simulink model "Modular_Model_New_Board_Enes"  (R2018a)
settings: Solver=VariableStepAuto  StartTime=0.0  StopTime=Tfinal  FixedStep=SampleTime*1e-2  MinStep=SampleTime*1e-2  RelTol=1e-3
values from neighbouring files (symbols this model uses):
  C1A = 5e-6    (= 5e-06)    [InverterMFile.m]    (also in sim_param_new_board.m)
  C1B = 5e-6    (= 5e-06)    [InverterMFile.m]    (also in sim_param_new_board.m)
  C1C = 5e-6    (= 5e-06)    [InverterMFile.m]    (also in sim_param_new_board.m)
  ESLA = 19e-15    (= 1.9e-14)    [sim_param_new_board.m]
  ESLB = 19e-15    (= 1.9e-14)    [sim_param_new_board.m]
  ESLC = 19e-15    (= 1.9e-14)    [sim_param_new_board.m]
  ESRA = 21.1e-15    (= 2.11e-14)    [sim_param_new_board.m]
  ESRB = 21.1e-15    (= 2.11e-14)    [sim_param_new_board.m]
  ESRC = 21.1e-15    (= 2.11e-14)    [sim_param_new_board.m]
  ffund = 50    [InverterMFile.m]    (also in mathematicalModelParam.m; sim_param_new_board.m)
  LABBot = 10.20e-9    (= 1.02e-08)    [sim_param_new_board.m]
  LABot = 20.25e-9    (= 2.025e-08)    [sim_param_new_board.m]
  LABTop = 18.30e-9    (= 1.83e-08)    [sim_param_new_board.m]
  LAMid = 01.30e-9    (= 1.3e-09)    [sim_param_new_board.m]
  LATop = 03.40e-9    (= 3.4e-09)    [sim_param_new_board.m]
  LBBot = 20.38e-9    (= 2.038e-08)    [sim_param_new_board.m]
  LBCBot = 11.14e-9    (= 1.114e-08)    [sim_param_new_board.m]
  LBCTop = 21.84e-9    (= 2.184e-08)    [sim_param_new_board.m]
  LBMid = 01.30e-9    (= 1.3e-09)    [sim_param_new_board.m]
  LBTop = 03.38e-9    (= 3.38e-09)    [sim_param_new_board.m]
  LCBot = 20.94e-9    (= 2.094e-08)    [sim_param_new_board.m]
  LCMid = 01.30e-9    (= 1.3e-09)    [sim_param_new_board.m]
  LCTop = 03.41e-9    (= 3.41e-09)    [sim_param_new_board.m]
  Ld = 0.9e-9    (= 9e-10)    [InverterMFile.m]    (also in sim_param_new_board.m)
  Lin = Lload1    [InverterMFile.m]    (also in sim_param_new_board.m)
  Lload1 = Xload1/(2*pi*ffund)    [InverterMFile.m]    (also in sim_param_new_board.m)
  Ls = 0.9e-9    (= 9e-10)    [InverterMFile.m]    (also in sim_param_new_board.m)
  ModulationIndex1 = 0.9    [InverterMFile.m]    (also in sim_param_new_board.m)
  Module1Phase = 0    [InverterMFile.m]    (also in sim_param_new_board.m)
  NEG1 = 100e-15    (= 1e-13)    [InverterMFile.m]    (also in sim_param_new_board.m)
  POS1 = 100e-15    (= 1e-13)    [InverterMFile.m]    (also in sim_param_new_board.m)
  RABBot = 10.20e-9    (= 1.02e-08)    [sim_param_new_board.m]
  RABot = 20.25e-9    (= 2.025e-08)    [sim_param_new_board.m]
  RABTop = 18.30e-9    (= 1.83e-08)    [sim_param_new_board.m]
  RAMid = 01.30e-9    (= 1.3e-09)    [sim_param_new_board.m]
  RATop = 03.40e-9    (= 3.4e-09)    [sim_param_new_board.m]
  RBBot = 20.38e-9    (= 2.038e-08)    [sim_param_new_board.m]
  RBCBot = 11.14e-9    (= 1.114e-08)    [sim_param_new_board.m]
  RBCTop = 21.84e-9    (= 2.184e-08)    [sim_param_new_board.m]
  RBMid = 01.30e-9    (= 1.3e-09)    [sim_param_new_board.m]
  RBTop = 03.38e-9    (= 3.38e-09)    [sim_param_new_board.m]
  RCBot = 20.94e-9    (= 2.094e-08)    [sim_param_new_board.m]
  RCMid = 01.30e-9    (= 1.3e-09)    [sim_param_new_board.m]
  RCTop = 03.41e-9    (= 3.41e-09)    [sim_param_new_board.m]
  Rin = 10    [InverterMFile.m]    (also in sim_param_new_board.m)
  Rload1 = Z1*PF    [InverterMFile.m]    (also in sim_param_new_board.m)
  Vin = Vdc + Idc*Rin    (= 418.148148148)    [InverterMFile.m]    (also in sim_param_new_board.m = 147.040202596)
  Vmodule = 270    [InverterMFile.m]    (also in sim_param_new_board.m)
  VpulseMax = 6    [InverterMFile.m]    (also in sim_param_new_board.m)
  VpulseMin = -3    [InverterMFile.m]    (also in sim_param_new_board.m)
libraries: powerlib x80, simulink x12, powerlib_meascontrol x4
settings Model: SimulationMode=accelerator  Creator=Furkan  LastModifiedBy=enes_
settings DataIOCC: SaveOutput=off  SignalLogging=off  DSMLogging=off  SaveTime=off
settings OptimizationCC: LifeSpan=inf
settings DebuggingCC: SFExecutionAtInitializationDiag=none
settings CodeAppCC: StateflowObjectComments=on
settings SimscapeCC: SimscapeNormalizeSystem=off

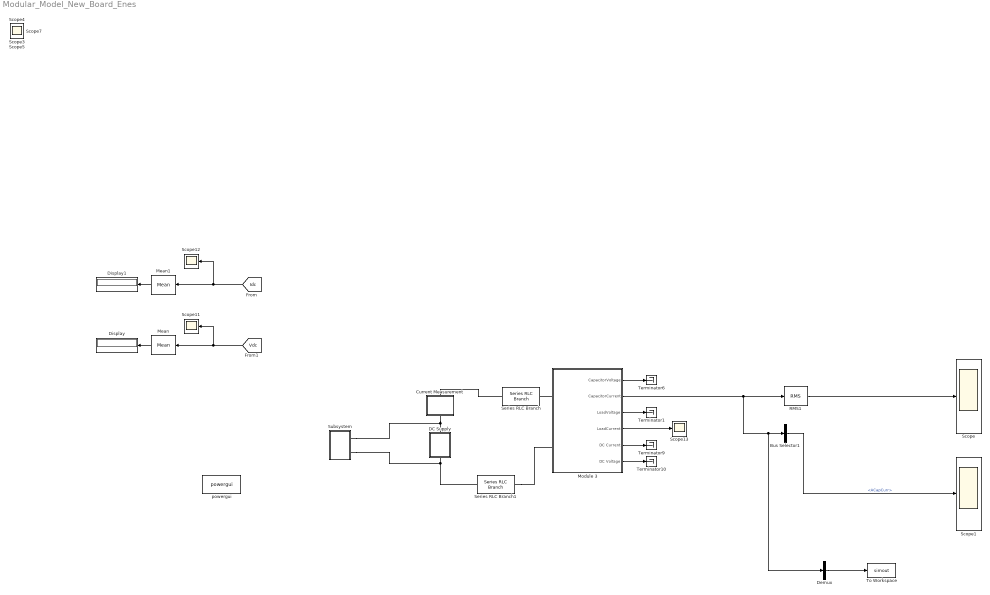
== system Modular_Model_New_Board_Enes ==
  Bus Selector1 : BusSelector  OutputSignals=ACapCurr
  Current Measurement : Subsystem
  DC Supply : Subsystem
  Demux : Demux  Outputs=3
  Display : Display
  Display1 : Display
  Mean : powerlib_meascontrol/Measurements/Mean  Freq=ffund  Vinit=0  Ts=0
  Mean1 : powerlib_meascontrol/Measurements/Mean  Freq=ffund  Vinit=0  Ts=0
  Module 3 : Subsystem
  RMS1 : powerlib_meascontrol/Measurements/RMS  TrueRMS=on  Freq=40000  RMSInit=0  Ts=0
  Scope : Scope  NumInputPorts=3
  Scope1 : Scope  NumInputPorts=3
  Scope{3..5,7,11..13} (7 alike) : Scope
  Series RLC Branch : powerlib/Elements/Series RLC Branch  LConnTagsString=__new0  RConnTagsString=__new0  BranchType=L  Resistance=1  Inductance=POS1  SetiL0=off  InitialCurrent=0  Capacitance=1e-6  Setx0=off  InitialVoltage=0  Measurements=None
  Series RLC Branch1 : powerlib/Elements/Series RLC Branch  LConnTagsString=__new0  RConnTagsString=__new0  BranchType=L  Resistance=1  Inductance=NEG1  SetiL0=off  InitialCurrent=0  Capacitance=1e-6  Setx0=off  InitialVoltage=0  Measurements=None
  Subsystem : Subsystem
  Terminator{1,6,9..10} (4 alike) : Terminator
  To Workspace : ToWorkspace  VariableName=simout  SaveFormat=Timeseries  SampleTime=-1
  powergui : powerlib/powergui  Priority=1  SimulationMode=Discrete  SampleTime=5e-6  frequency=60  Iterations=50  frequencyindice=0  Pbase=100e6  ErrMax=1e-4  UnitsV=kV  UnitsW=MW  buscounter=0  FunctionMessages=off  echomessages=off  EnableUseOfTLC=off  CurrentSourceSwitches=off  DisableSnubberDevices=off  DisableRonSwitches=off  DisableVfSwitches=off  DisplayEquations=off  SolverType=Tustin/Backward Euler (TBE)  Interpol=off  ExternalGateDelay=off  methode=off  Ts=100  x0status=blocks  SPID=off  SwTol=0  HookPort=off  RestoreLinks=warning  ResistiveCurrentMeasurement=off  Frange=[0:2:500]  Ylog=off  Xlog=on  ShowGrid=off  save=off  variable=ZData  structure=0  ZoomFFT=off  StartTime=0.0  cycles=1  DisplayStyle=1  fundamental=60  FreqAxis=off  MaxFrequency=1000  frequencyindicesteady=1  RmsSteady=1  display=off
  wires:
  [Vdc] -> Mean/1, Scope11/1
  [Idc] -> Mean1/1, Scope12/1
  Module 3/1(CapacitorVoltage) -> Terminator6/1
  Module 3/2(CapacitorCurrent) -> Demux/1, Bus Selector1/1, RMS1/1
  Module 3/5(DC Current) -> Terminator9/1
  Module 3/6(DC Voltage) -> Terminator10/1
  RMS1/1 -> Scope/2
  Bus Selector1/1 -> Scope1/2  "<ACapCurr>"
  Mean/1 -> Display/1
  Mean1/1 -> Display1/1
  Module 3/3(LoadVoltage) -> Terminator1/1
  Module 3/4(LoadCurrent) -> Scope13/1
  Demux/2 -> To Workspace/1
  connections:
  DC Supply/LConn1 -- Series RLC Branch1/LConn1 -- Subsystem/LConn2
  Current Measurement/RConn1 -- DC Supply/RConn1 -- Subsystem/LConn1
  Module 3/LConn1 -- Series RLC Branch/RConn1
  Current Measurement/LConn1 -- Series RLC Branch/LConn1
  Series RLC Branch1/RConn1 -- Module 3/LConn2

== system Modular_Model_New_Board_Enes/Current Measurement ==
  Current Measurement : powerlib/Measurements/Current Measurement  PhasorSimulation=off  OutputType=Complex  PSBequivalent=0
  DC+ : PMIOPort  Side=Left
  i+ : PMIOPort  Port=2  Side=Right
  tag scope: Idc=global
  wires:
  Current Measurement/1 -> [Idc]
  connections:
  DC+/RConn1 -- Current Measurement/RConn1
  Current Measurement/LConn1 -- i+/RConn1

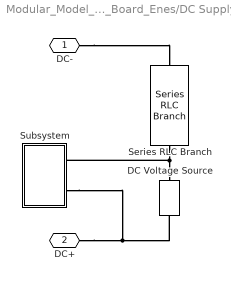
== system Modular_Model_New_Board_Enes/DC Supply ==
  DC Voltage Source : powerlib/Electrical Sources/DC Voltage Source  Amplitude=Vin  Measurements=None
  Series RLC Branch : powerlib/Elements/Series RLC Branch  LConnTagsString=__new0  RConnTagsString=__new0  BranchType=RL  Resistance=Rin  Inductance=Lin  SetiL0=off  InitialCurrent=0  Capacitance=1e-6  Setx0=off  InitialVoltage=0  Measurements=None
  Subsystem : Subsystem
  DC- : PMIOPort  Side=Left
  DC+ : PMIOPort  Port=2  Side=Right
  connections:
  DC-/RConn1 -- Series RLC Branch/RConn1
  DC+/RConn1 -- Subsystem/LConn2 -- DC Voltage Source/RConn1
  Series RLC Branch/LConn1 -- DC Voltage Source/LConn1 -- Subsystem/LConn1

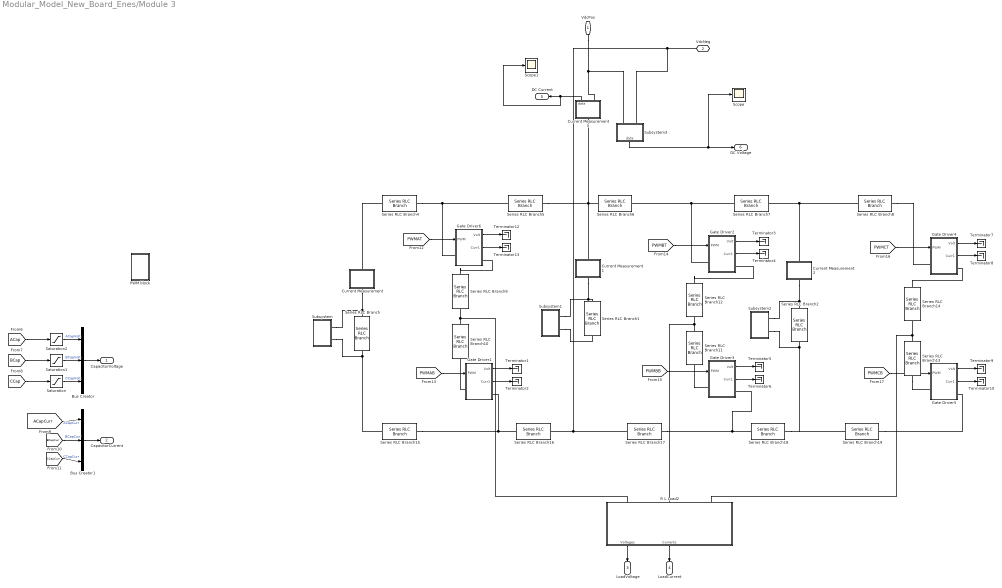
== system Modular_Model_New_Board_Enes/Module 3 ==
  Bus Creator : BusCreator  Inputs=3
  Bus Creator1 : BusCreator  Inputs=3
  Current Measurement : Subsystem
  Current Measurement1 : Subsystem
  Current Measurement2 : Subsystem
  Current Measurement3 : Subsystem
  Gate Driver1 : Subsystem
  Gate Driver2 : Subsystem
  Gate Driver3 : Subsystem
  Gate Driver4 : Subsystem
  Gate Driver5 : Subsystem
  Gate Driver6 : Subsystem
  PWM block : Subsystem
  R L Load2 : Subsystem
  Saturation : Saturate  UpperLimit=Vmodule*1.5  LowerLimit=-20
  Saturation1 : Saturate  UpperLimit=Vmodule*1.5  LowerLimit=-20
  Saturation2 : Saturate  UpperLimit=Vmodule*1.5  LowerLimit=-20
  Scope : Scope
  Scope1 : Scope
  Series RLC Branch : powerlib/Elements/Series RLC Branch  LConnTagsString=__new0  RConnTagsString=__new0  BranchType=RLC  Resistance=ESRA  Inductance=ESLA  SetiL0=off  InitialCurrent=0  Capacitance=C1A  Setx0=on  InitialVoltage=Vdc  Measurements=None
  Series RLC Branch1 : powerlib/Elements/Series RLC Branch  LConnTagsString=__new0  RConnTagsString=__new0  BranchType=RLC  Resistance=ESRB  Inductance=ESLB  SetiL0=off  InitialCurrent=0  Capacitance=C1B  Setx0=on  InitialVoltage=Vdc  Measurements=None
  Series RLC Branch10 : powerlib/Elements/Series RLC Branch  LConnTagsString=__new0  RConnTagsString=__new0  BranchType=RL  Resistance=RAMid/2  Inductance=LAMid/2  SetiL0=off  InitialCurrent=0  Capacitance=1e-6  Setx0=off  InitialVoltage=0  Measurements=None
  Series RLC Branch11 : powerlib/Elements/Series RLC Branch  LConnTagsString=__new0  RConnTagsString=__new0  BranchType=RL  Resistance=RBMid/2  Inductance=LBMid/2  SetiL0=off  InitialCurrent=0  Capacitance=1e-6  Setx0=off  InitialVoltage=0  Measurements=None
  Series RLC Branch12 : powerlib/Elements/Series RLC Branch  LConnTagsString=__new0  RConnTagsString=__new0  BranchType=RL  Resistance=RBMid/2  Inductance=LBMid/2  SetiL0=off  InitialCurrent=0  Capacitance=1e-6  Setx0=off  InitialVoltage=0  Measurements=None
  Series RLC Branch13 : powerlib/Elements/Series RLC Branch  LConnTagsString=__new0  RConnTagsString=__new0  BranchType=RL  Resistance=RCMid/2  Inductance=LCMid/2  SetiL0=off  InitialCurrent=0  Capacitance=1e-6  Setx0=off  InitialVoltage=0  Measurements=None
  Series RLC Branch14 : powerlib/Elements/Series RLC Branch  LConnTagsString=__new0  RConnTagsString=__new0  BranchType=RL  Resistance=RCMid/2  Inductance=LCMid/2  SetiL0=off  InitialCurrent=0  Capacitance=1e-6  Setx0=off  InitialVoltage=0  Measurements=None
  Series RLC Branch15 : powerlib/Elements/Series RLC Branch  LConnTagsString=__new0  RConnTagsString=__new0  BranchType=RL  Resistance=RABot  Inductance=LABot  SetiL0=off  InitialCurrent=0  Capacitance=1e-6  Setx0=off  InitialVoltage=0  Measurements=None
  Series RLC Branch16 : powerlib/Elements/Series RLC Branch  LConnTagsString=__new0  RConnTagsString=__new0  BranchType=RL  Resistance=RABBot  Inductance=LABBot  SetiL0=off  InitialCurrent=0  Capacitance=1e-6  Setx0=off  InitialVoltage=0  Measurements=None
  Series RLC Branch17 : powerlib/Elements/Series RLC Branch  LConnTagsString=__new0  RConnTagsString=__new0  BranchType=RL  Resistance=RBBot  Inductance=LBBot  SetiL0=off  InitialCurrent=0  Capacitance=1e-6  Setx0=off  InitialVoltage=0  Measurements=None
  Series RLC Branch18 : powerlib/Elements/Series RLC Branch  LConnTagsString=__new0  RConnTagsString=__new0  BranchType=RL  Resistance=RBCBot  Inductance=LBCBot  SetiL0=off  InitialCurrent=0  Capacitance=1e-6  Setx0=off  InitialVoltage=0  Measurements=None
  Series RLC Branch19 : powerlib/Elements/Series RLC Branch  LConnTagsString=__new0  RConnTagsString=__new0  BranchType=RL  Resistance=RCBot  Inductance=LCBot  SetiL0=off  InitialCurrent=0  Capacitance=1e-6  Setx0=off  InitialVoltage=0  Measurements=None
  Series RLC Branch2 : powerlib/Elements/Series RLC Branch  LConnTagsString=__new0  RConnTagsString=__new0  BranchType=RLC  Resistance=ESRC  Inductance=ESLC  SetiL0=off  InitialCurrent=0  Capacitance=C1C  Setx0=on  InitialVoltage=Vdc  Measurements=None
  Series RLC Branch4 : powerlib/Elements/Series RLC Branch  LConnTagsString=__new0  RConnTagsString=__new0  BranchType=RL  Resistance=RATop  Inductance=LATop  SetiL0=off  InitialCurrent=0  Capacitance=1e-6  Setx0=off  InitialVoltage=0  Measurements=None
  Series RLC Branch5 : powerlib/Elements/Series RLC Branch  LConnTagsString=__new0  RConnTagsString=__new0  BranchType=RL  Resistance=RABTop  Inductance=LABTop  SetiL0=off  InitialCurrent=0  Capacitance=1e-6  Setx0=off  InitialVoltage=0  Measurements=None
  Series RLC Branch6 : powerlib/Elements/Series RLC Branch  LConnTagsString=__new0  RConnTagsString=__new0  BranchType=RL  Resistance=RBTop  Inductance=LBTop  SetiL0=off  InitialCurrent=0  Capacitance=1e-6  Setx0=off  InitialVoltage=0  Measurements=None
  Series RLC Branch7 : powerlib/Elements/Series RLC Branch  LConnTagsString=__new0  RConnTagsString=__new0  BranchType=RL  Resistance=RBCTop  Inductance=LBCTop  SetiL0=off  InitialCurrent=0  Capacitance=1e-6  Setx0=off  InitialVoltage=0  Measurements=None
  Series RLC Branch8 : powerlib/Elements/Series RLC Branch  LConnTagsString=__new0  RConnTagsString=__new0  BranchType=RL  Resistance=RCTop  Inductance=LCTop  SetiL0=off  InitialCurrent=0  Capacitance=1e-6  Setx0=off  InitialVoltage=0  Measurements=None
  Series RLC Branch9 : powerlib/Elements/Series RLC Branch  LConnTagsString=__new0  RConnTagsString=__new0  BranchType=RL  Resistance=RAMid/2  Inductance=LAMid/2  SetiL0=off  InitialCurrent=0  Capacitance=1e-6  Setx0=off  InitialVoltage=0  Measurements=None
  Subsystem : Subsystem
  Subsystem1 : Subsystem
  Subsystem2 : Subsystem
  Subsystem3 : Subsystem
  Terminator{1..10,12..13} (12 alike) : Terminator
  VdcPos : PMIOPort  Side=Left
  VdcNeg : PMIOPort  Port=2  Side=Left
  CapacitorVoltage : Outport
  CapacitorCurrent : Outport  Port=2
  LoadVoltage : Outport  Port=3
  LoadCurrent : Outport  Port=4
  DC Current : Outport  Port=5
  DC Voltage : Outport  Port=6
  wires:
  [ACap] -> Saturation2/1
  [BCap] -> Saturation1/1
  [CCap] -> Saturation/1
  Bus Creator/1 -> CapacitorVoltage/1
  [CCapCurr] -> Bus Creator1/3  "CCapCurr"
  [BCapCurr] -> Bus Creator1/2  "BCapCurr"
  [ACapCurr] -> Bus Creator1/1  "ACapCurr"
  Bus Creator1/1 -> CapacitorCurrent/1
  Saturation/1 -> Bus Creator/3  "CCapVolt"
  Saturation1/1 -> Bus Creator/2  "BCapVolt"
  Saturation2/1 -> Bus Creator/1  "ACapVolt"
  [PWMAT] -> Gate Driver6/1(PWM)
  Gate Driver6/1(Volt) -> Terminator12/1
  Gate Driver6/2(Curr1) -> Terminator13/1
  R L Load2/2(Currents) -> LoadCurrent/1
  R L Load2/1(Voltages) -> LoadVoltage/1
  Current Measurement3/1(data) -> Scope1/1, DC Current/1
  Subsystem3/1(data) -> Scope/1, DC Voltage/1
  Gate Driver1/1(Volt) -> Terminator1/1
  Gate Driver1/2(Curr1) -> Terminator2/1
  [PWMAB] -> Gate Driver1/1(PWM)
  Gate Driver2/1(Volt) -> Terminator3/1
  Gate Driver2/2(Curr1) -> Terminator4/1
  [PWMBT] -> Gate Driver2/1(PWM)
  Gate Driver3/1(Volt) -> Terminator5/1
  Gate Driver3/2(Curr1) -> Terminator6/1
  [PWMBB] -> Gate Driver3/1(PWM)
  Gate Driver4/1(Volt) -> Terminator7/1
  Gate Driver4/2(Curr1) -> Terminator8/1
  [PWMCT] -> Gate Driver4/1(PWM)
  Gate Driver5/1(Volt) -> Terminator9/1
  Gate Driver5/2(Curr1) -> Terminator10/1
  [PWMCB] -> Gate Driver5/1(PWM)
  connections:
  Subsystem/LConn1 -- Series RLC Branch/LConn1 -- Current Measurement/LConn1
  Subsystem/LConn2 -- Series RLC Branch/RConn1 -- Series RLC Branch15/LConn1
  Subsystem1/LConn1 -- Series RLC Branch1/LConn1 -- Current Measurement1/LConn1
  Subsystem1/LConn2 -- Series RLC Branch1/RConn1
  Subsystem2/LConn1 -- Series RLC Branch2/LConn1 -- Current Measurement2/LConn1
  Subsystem2/LConn2 -- Series RLC Branch2/RConn1 -- Series RLC Branch19/LConn1 -- Series RLC Branch18/RConn1
  Series RLC Branch4/LConn1 -- Current Measurement/RConn1
  Series RLC Branch4/RConn1 -- Series RLC Branch5/LConn1 -- Gate Driver6/LConn1
  Gate Driver2/LConn1 -- Series RLC Branch6/RConn1 -- Series RLC Branch7/LConn1
  Current Measurement2/RConn1 -- Series RLC Branch7/RConn1 -- Series RLC Branch8/LConn1
  Series RLC Branch8/RConn1 -- Gate Driver4/LConn1
  Series RLC Branch10/LConn1 -- R L Load2/LConn1 -- Series RLC Branch9/RConn1
  Gate Driver1/LConn1 -- Series RLC Branch10/RConn1
  Series RLC Branch9/LConn1 -- Gate Driver6/RConn1
  Series RLC Branch11/LConn1 -- R L Load2/LConn2 -- Series RLC Branch12/RConn1
  Series RLC Branch11/RConn1 -- Gate Driver3/LConn1
  Series RLC Branch12/LConn1 -- Gate Driver2/RConn1
  Series RLC Branch13/LConn1 -- R L Load2/LConn3 -- Series RLC Branch14/RConn1
  Series RLC Branch14/LConn1 -- Gate Driver4/RConn1
  Series RLC Branch13/RConn1 -- Gate Driver5/LConn1
  Series RLC Branch15/RConn1 -- Series RLC Branch16/LConn1 -- Gate Driver1/RConn1
  Series RLC Branch17/RConn1 -- Series RLC Branch18/LConn1 -- Gate Driver3/RConn1
  Series RLC Branch19/RConn1 -- Gate Driver5/RConn1
  Series RLC Branch5/RConn1 -- Series RLC Branch6/LConn1 -- Current Measurement3/LConn1 -- Current Measurement1/RConn1
  Series RLC Branch17/LConn1 -- Subsystem3/LConn2 -- VdcNeg/RConn1 -- Series RLC Branch16/RConn1
  Current Measurement3/RConn1 -- Subsystem3/LConn1 -- VdcPos/RConn1

== system Modular_Model_New_Board_Enes/Subsystem ==
  Voltage Measurement : powerlib/Measurements/Voltage Measurement  PhasorSimulation=off  OutputType=Complex  PSBequivalent=0
  V+ : PMIOPort  Side=Left
  V- : PMIOPort  Port=2  Side=Left
  tag scope: Vdc=global
  wires:
  Voltage Measurement/1 -> [Vdc]
  connections:
  Voltage Measurement/LConn1 -- V+/RConn1
  Voltage Measurement/LConn2 -- V-/RConn1

== system Modular_Model_New_Board_Enes/DC Supply/Subsystem ==
  Scope : Scope
  Voltage Measurement : powerlib/Measurements/Voltage Measurement  PhasorSimulation=off  OutputType=Complex  PSBequivalent=0
  V+ : PMIOPort  Side=Left
  V- : PMIOPort  Port=2  Side=Left
  wires:
  Voltage Measurement/1 -> Scope/1
  connections:
  Voltage Measurement/LConn1 -- V+/RConn1
  Voltage Measurement/LConn2 -- V-/RConn1

== system Modular_Model_New_Board_Enes/Module 3/Current Measurement ==
  Current Measurement : powerlib/Measurements/Current Measurement  PhasorSimulation=off  OutputType=Complex  PSBequivalent=0
  i- : PMIOPort  Side=Left
  i+ : PMIOPort  Port=2  Side=Right
  tag scope: ACapCurr=global
  wires:
  Current Measurement/1 -> [ACapCurr]
  connections:
  i-/RConn1 -- Current Measurement/RConn1
  Current Measurement/LConn1 -- i+/RConn1

== system Modular_Model_New_Board_Enes/Module 3/Current Measurement1 ==
  Current Measurement : powerlib/Measurements/Current Measurement  PhasorSimulation=off  OutputType=Complex  PSBequivalent=0
  i- : PMIOPort  Side=Left
  i+ : PMIOPort  Port=2  Side=Right
  tag scope: BCapCurr=global
  wires:
  Current Measurement/1 -> [BCapCurr]
  connections:
  i-/RConn1 -- Current Measurement/RConn1
  Current Measurement/LConn1 -- i+/RConn1

== system Modular_Model_New_Board_Enes/Module 3/Current Measurement2 ==
  Current Measurement : powerlib/Measurements/Current Measurement  PhasorSimulation=off  OutputType=Complex  PSBequivalent=0
  i- : PMIOPort  Side=Left
  i+ : PMIOPort  Port=2  Side=Right
  tag scope: CCapCurr=global
  wires:
  Current Measurement/1 -> [CCapCurr]
  connections:
  i-/RConn1 -- Current Measurement/RConn1
  Current Measurement/LConn1 -- i+/RConn1

== system Modular_Model_New_Board_Enes/Module 3/Current Measurement3 ==
  Current Measurement : powerlib/Measurements/Current Measurement  PhasorSimulation=off  OutputType=Complex  PSBequivalent=0
  i- : PMIOPort  Side=Left
  i+ : PMIOPort  Port=2  Side=Right
  data : Outport
  wires:
  Current Measurement/1 -> data/1
  connections:
  i-/RConn1 -- Current Measurement/RConn1
  Current Measurement/LConn1 -- i+/RConn1

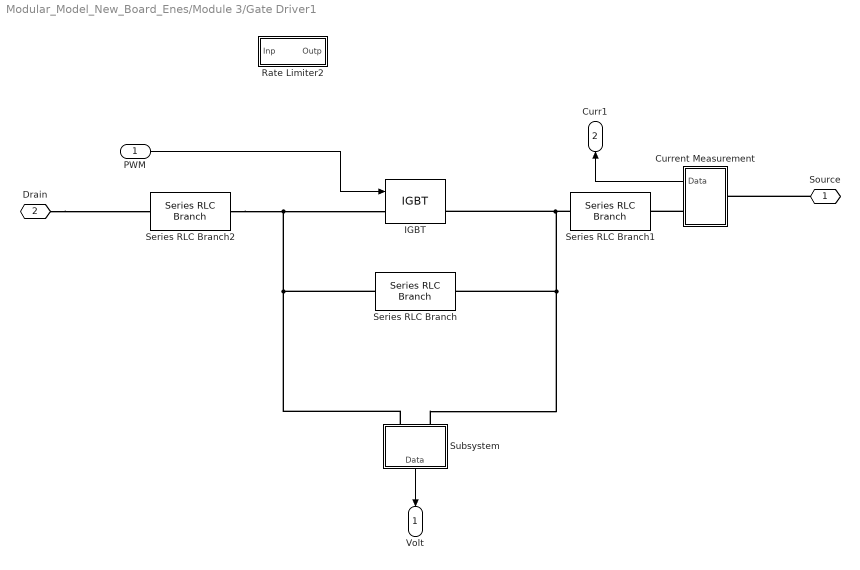
== system Modular_Model_New_Board_Enes/Module 3/Gate Driver1 ==
  PWM : Inport
  Current Measurement : Subsystem
  IGBT : powerlib/Power Electronics/IGBT  Ron=0.001  Lon=0  Vf=1  Tf=1e-6  Tt=2e-6  IC=0  Rs=1e5  Cs=inf  Measurements=on
  Rate Limiter2 : Subsystem
  Series RLC Branch : powerlib/Elements/Series RLC Branch  LConnTagsString=__new0  RConnTagsString=__new0  BranchType=C  Resistance=1  Inductance=1e-3  SetiL0=off  InitialCurrent=0  Capacitance=142e-12  Setx0=off  InitialVoltage=0  Measurements=None
  Series RLC Branch1 : powerlib/Elements/Series RLC Branch  LConnTagsString=__new0  RConnTagsString=__new0  BranchType=L  Resistance=1  Inductance=Ls  SetiL0=off  InitialCurrent=0  Capacitance=1e-6  Setx0=off  InitialVoltage=0  Measurements=None
  Series RLC Branch2 : powerlib/Elements/Series RLC Branch  LConnTagsString=__new0  RConnTagsString=__new0  BranchType=L  Resistance=1  Inductance=Ld  SetiL0=off  InitialCurrent=0  Capacitance=1e-6  Setx0=off  InitialVoltage=0  Measurements=None
  Subsystem : Subsystem
  Source : PMIOPort  Side=Right
  Drain : PMIOPort  Port=2  Side=Left
  Volt : Outport
  Curr1 : Outport  Port=2
  wires:
  PWM/1 -> IGBT/1
  Subsystem/1(Data) -> Volt/1
  Current Measurement/1(Data) -> Curr1/1
  connections:
  Series RLC Branch/LConn1 -- Subsystem/LConn1 -- IGBT/LConn1 -- Series RLC Branch2/RConn1
  Subsystem/LConn2 -- Series RLC Branch/RConn1 -- Series RLC Branch1/LConn1 -- IGBT/RConn1
  Source/RConn1 -- Current Measurement/LConn1
  Drain/RConn1 -- Series RLC Branch2/LConn1
  Current Measurement/RConn1 -- Series RLC Branch1/RConn1

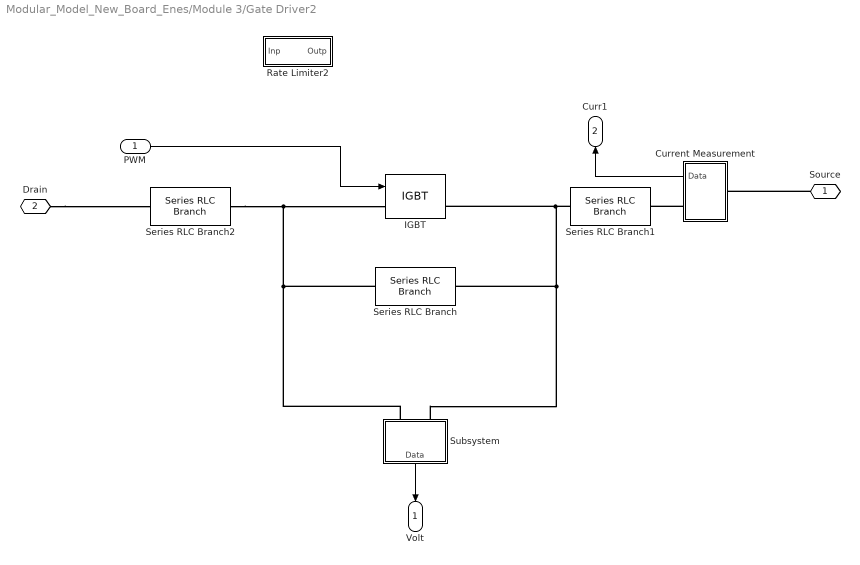
== system Modular_Model_New_Board_Enes/Module 3/Gate Driver2 ==
  PWM : Inport
  Current Measurement : Subsystem
  IGBT : powerlib/Power Electronics/IGBT  Ron=0.001  Lon=0  Vf=1  Tf=1e-6  Tt=2e-6  IC=0  Rs=1e5  Cs=inf  Measurements=on
  Rate Limiter2 : Subsystem
  Series RLC Branch : powerlib/Elements/Series RLC Branch  LConnTagsString=__new0  RConnTagsString=__new0  BranchType=C  Resistance=1  Inductance=1e-3  SetiL0=off  InitialCurrent=0  Capacitance=142e-12  Setx0=off  InitialVoltage=0  Measurements=None
  Series RLC Branch1 : powerlib/Elements/Series RLC Branch  LConnTagsString=__new0  RConnTagsString=__new0  BranchType=L  Resistance=1  Inductance=Ls  SetiL0=off  InitialCurrent=0  Capacitance=1e-6  Setx0=off  InitialVoltage=0  Measurements=None
  Series RLC Branch2 : powerlib/Elements/Series RLC Branch  LConnTagsString=__new0  RConnTagsString=__new0  BranchType=L  Resistance=1  Inductance=Ld  SetiL0=off  InitialCurrent=0  Capacitance=1e-6  Setx0=off  InitialVoltage=0  Measurements=None
  Subsystem : Subsystem
  Source : PMIOPort  Side=Right
  Drain : PMIOPort  Port=2  Side=Left
  Volt : Outport
  Curr1 : Outport  Port=2
  wires:
  PWM/1 -> IGBT/1
  Subsystem/1(Data) -> Volt/1
  Current Measurement/1(Data) -> Curr1/1
  connections:
  Series RLC Branch/LConn1 -- Subsystem/LConn1 -- IGBT/LConn1 -- Series RLC Branch2/RConn1
  Subsystem/LConn2 -- Series RLC Branch/RConn1 -- Series RLC Branch1/LConn1 -- IGBT/RConn1
  Source/RConn1 -- Current Measurement/LConn1
  Drain/RConn1 -- Series RLC Branch2/LConn1
  Current Measurement/RConn1 -- Series RLC Branch1/RConn1

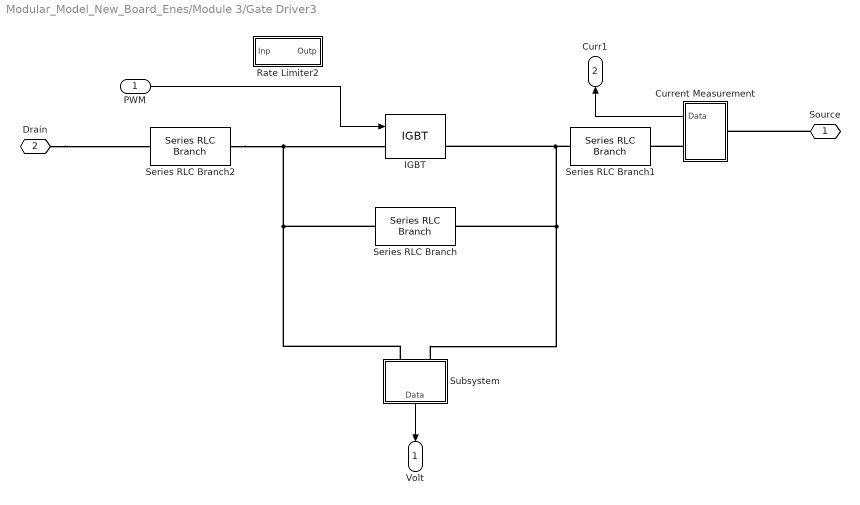
== system Modular_Model_New_Board_Enes/Module 3/Gate Driver3 ==
  PWM : Inport
  Current Measurement : Subsystem
  IGBT : powerlib/Power Electronics/IGBT  Ron=0.001  Lon=0  Vf=1  Tf=1e-6  Tt=2e-6  IC=0  Rs=1e5  Cs=inf  Measurements=on
  Rate Limiter2 : Subsystem
  Series RLC Branch : powerlib/Elements/Series RLC Branch  LConnTagsString=__new0  RConnTagsString=__new0  BranchType=C  Resistance=1  Inductance=1e-3  SetiL0=off  InitialCurrent=0  Capacitance=142e-12  Setx0=off  InitialVoltage=0  Measurements=None
  Series RLC Branch1 : powerlib/Elements/Series RLC Branch  LConnTagsString=__new0  RConnTagsString=__new0  BranchType=L  Resistance=1  Inductance=Ls  SetiL0=off  InitialCurrent=0  Capacitance=1e-6  Setx0=off  InitialVoltage=0  Measurements=None
  Series RLC Branch2 : powerlib/Elements/Series RLC Branch  LConnTagsString=__new0  RConnTagsString=__new0  BranchType=L  Resistance=1  Inductance=Ld  SetiL0=off  InitialCurrent=0  Capacitance=1e-6  Setx0=off  InitialVoltage=0  Measurements=None
  Subsystem : Subsystem
  Source : PMIOPort  Side=Right
  Drain : PMIOPort  Port=2  Side=Left
  Volt : Outport
  Curr1 : Outport  Port=2
  wires:
  PWM/1 -> IGBT/1
  Subsystem/1(Data) -> Volt/1
  Current Measurement/1(Data) -> Curr1/1
  connections:
  Series RLC Branch/LConn1 -- Subsystem/LConn1 -- IGBT/LConn1 -- Series RLC Branch2/RConn1
  Source/RConn1 -- Current Measurement/LConn1
  Drain/RConn1 -- Series RLC Branch2/LConn1
  Current Measurement/RConn1 -- Series RLC Branch1/RConn1
  Subsystem/LConn2 -- Series RLC Branch/RConn1 -- Series RLC Branch1/LConn1 -- IGBT/RConn1

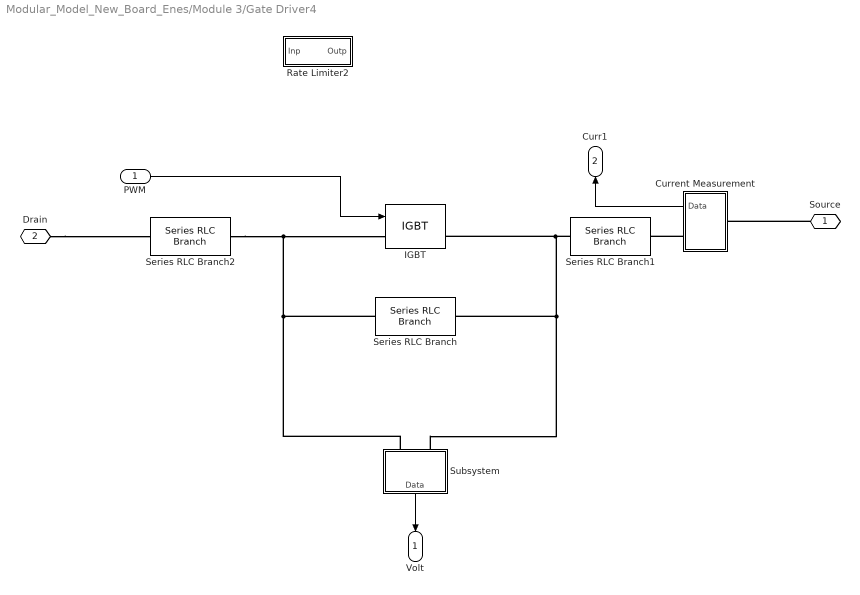
== system Modular_Model_New_Board_Enes/Module 3/Gate Driver4 ==
  PWM : Inport
  Current Measurement : Subsystem
  IGBT : powerlib/Power Electronics/IGBT  Ron=0.001  Lon=0  Vf=1  Tf=1e-6  Tt=2e-6  IC=0  Rs=1e5  Cs=inf  Measurements=on
  Rate Limiter2 : Subsystem
  Series RLC Branch : powerlib/Elements/Series RLC Branch  LConnTagsString=__new0  RConnTagsString=__new0  BranchType=C  Resistance=1  Inductance=1e-3  SetiL0=off  InitialCurrent=0  Capacitance=142e-12  Setx0=off  InitialVoltage=0  Measurements=None
  Series RLC Branch1 : powerlib/Elements/Series RLC Branch  LConnTagsString=__new0  RConnTagsString=__new0  BranchType=L  Resistance=1  Inductance=Ls  SetiL0=off  InitialCurrent=0  Capacitance=1e-6  Setx0=off  InitialVoltage=0  Measurements=None
  Series RLC Branch2 : powerlib/Elements/Series RLC Branch  LConnTagsString=__new0  RConnTagsString=__new0  BranchType=L  Resistance=1  Inductance=Ld  SetiL0=off  InitialCurrent=0  Capacitance=1e-6  Setx0=off  InitialVoltage=0  Measurements=None
  Subsystem : Subsystem
  Source : PMIOPort  Side=Right
  Drain : PMIOPort  Port=2  Side=Left
  Volt : Outport
  Curr1 : Outport  Port=2
  wires:
  PWM/1 -> IGBT/1
  Subsystem/1(Data) -> Volt/1
  Current Measurement/1(Data) -> Curr1/1
  connections:
  Series RLC Branch/LConn1 -- Subsystem/LConn1 -- IGBT/LConn1 -- Series RLC Branch2/RConn1
  Subsystem/LConn2 -- Series RLC Branch/RConn1 -- Series RLC Branch1/LConn1 -- IGBT/RConn1
  Source/RConn1 -- Current Measurement/LConn1
  Drain/RConn1 -- Series RLC Branch2/LConn1
  Current Measurement/RConn1 -- Series RLC Branch1/RConn1

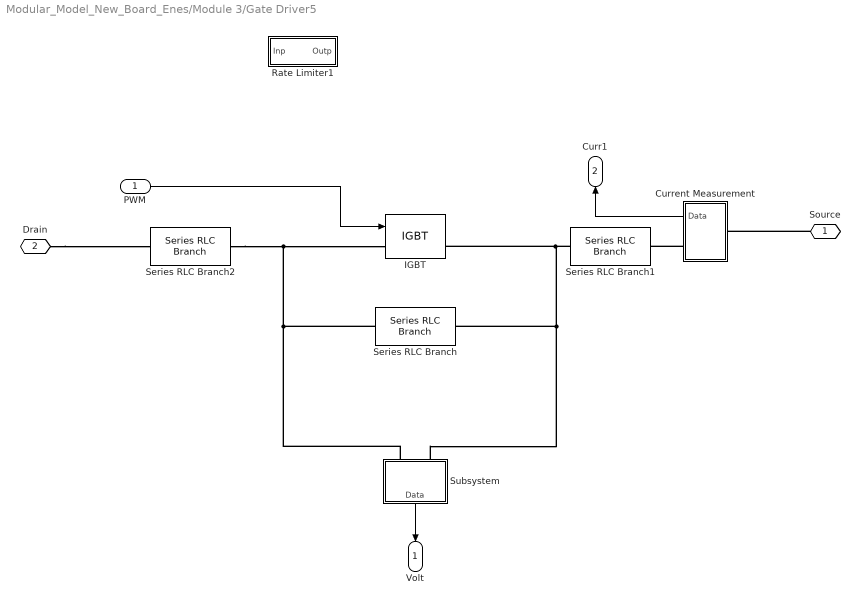
== system Modular_Model_New_Board_Enes/Module 3/Gate Driver5 ==
  PWM : Inport
  Current Measurement : Subsystem
  IGBT : powerlib/Power Electronics/IGBT  Ron=0.001  Lon=0  Vf=1  Tf=1e-6  Tt=2e-6  IC=0  Rs=1e5  Cs=inf  Measurements=on
  Rate Limiter1 : Subsystem
  Series RLC Branch : powerlib/Elements/Series RLC Branch  LConnTagsString=__new0  RConnTagsString=__new0  BranchType=C  Resistance=1  Inductance=1e-3  SetiL0=off  InitialCurrent=0  Capacitance=142e-12  Setx0=off  InitialVoltage=0  Measurements=None
  Series RLC Branch1 : powerlib/Elements/Series RLC Branch  LConnTagsString=__new0  RConnTagsString=__new0  BranchType=L  Resistance=1  Inductance=Ls  SetiL0=off  InitialCurrent=0  Capacitance=1e-6  Setx0=off  InitialVoltage=0  Measurements=None
  Series RLC Branch2 : powerlib/Elements/Series RLC Branch  LConnTagsString=__new0  RConnTagsString=__new0  BranchType=L  Resistance=1  Inductance=Ld  SetiL0=off  InitialCurrent=0  Capacitance=1e-6  Setx0=off  InitialVoltage=0  Measurements=None
  Subsystem : Subsystem
  Source : PMIOPort  Side=Right
  Drain : PMIOPort  Port=2  Side=Left
  Volt : Outport
  Curr1 : Outport  Port=2
  wires:
  PWM/1 -> IGBT/1
  Subsystem/1(Data) -> Volt/1
  Current Measurement/1(Data) -> Curr1/1
  connections:
  Series RLC Branch/LConn1 -- Subsystem/LConn1 -- IGBT/LConn1 -- Series RLC Branch2/RConn1
  Subsystem/LConn2 -- Series RLC Branch/RConn1 -- Series RLC Branch1/LConn1 -- IGBT/RConn1
  Source/RConn1 -- Current Measurement/LConn1
  Drain/RConn1 -- Series RLC Branch2/LConn1
  Current Measurement/RConn1 -- Series RLC Branch1/RConn1

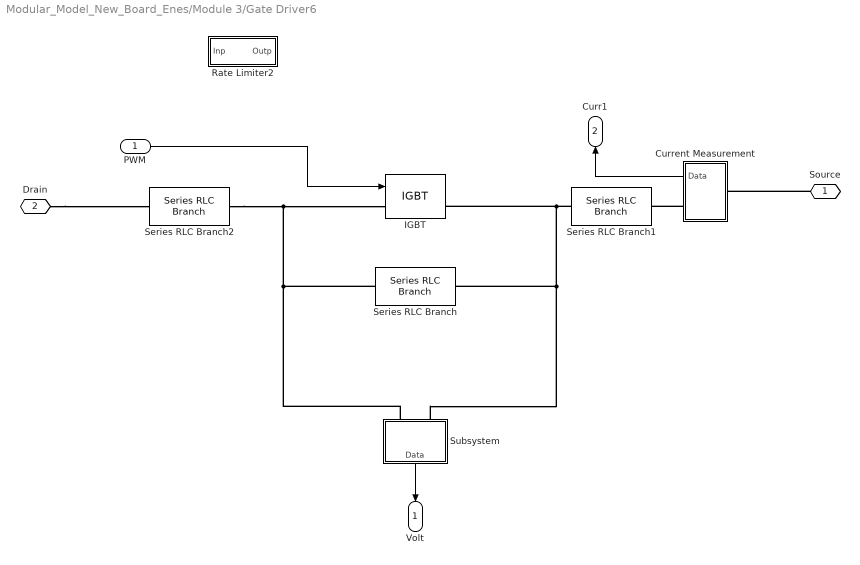
== system Modular_Model_New_Board_Enes/Module 3/Gate Driver6 ==
  PWM : Inport
  Current Measurement : Subsystem
  IGBT : powerlib/Power Electronics/IGBT  Ron=0.001  Lon=0  Vf=1  Tf=1e-6  Tt=2e-6  IC=0  Rs=1e5  Cs=inf  Measurements=on
  Rate Limiter2 : Subsystem
  Series RLC Branch : powerlib/Elements/Series RLC Branch  LConnTagsString=__new0  RConnTagsString=__new0  BranchType=C  Resistance=1  Inductance=1e-3  SetiL0=off  InitialCurrent=0  Capacitance=142e-12  Setx0=off  InitialVoltage=0  Measurements=None
  Series RLC Branch1 : powerlib/Elements/Series RLC Branch  LConnTagsString=__new0  RConnTagsString=__new0  BranchType=L  Resistance=1  Inductance=Ls  SetiL0=off  InitialCurrent=0  Capacitance=1e-6  Setx0=off  InitialVoltage=0  Measurements=None
  Series RLC Branch2 : powerlib/Elements/Series RLC Branch  LConnTagsString=__new0  RConnTagsString=__new0  BranchType=L  Resistance=1  Inductance=Ld  SetiL0=off  InitialCurrent=0  Capacitance=1e-6  Setx0=off  InitialVoltage=0  Measurements=None
  Subsystem : Subsystem
  Source : PMIOPort  Side=Right
  Drain : PMIOPort  Port=2  Side=Left
  Volt : Outport
  Curr1 : Outport  Port=2
  wires:
  PWM/1 -> IGBT/1
  Subsystem/1(Data) -> Volt/1
  Current Measurement/1(Data) -> Curr1/1
  connections:
  Subsystem/LConn1 -- Series RLC Branch2/RConn1 -- IGBT/LConn1 -- Series RLC Branch/LConn1
  Subsystem/LConn2 -- Series RLC Branch1/LConn1 -- IGBT/RConn1 -- Series RLC Branch/RConn1
  Source/RConn1 -- Current Measurement/LConn1
  Drain/RConn1 -- Series RLC Branch2/LConn1
  Current Measurement/RConn1 -- Series RLC Branch1/RConn1

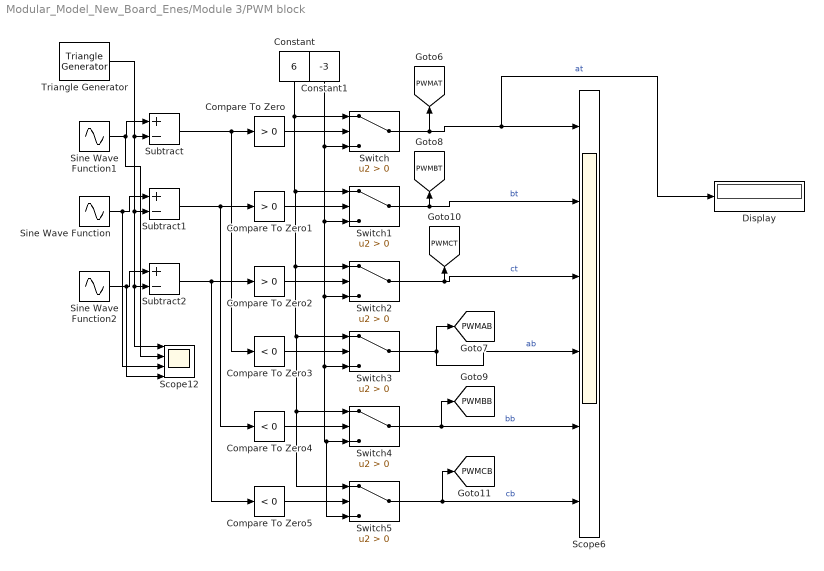
== system Modular_Model_New_Board_Enes/Module 3/PWM block ==
  Compare To Zero : simulink/Logic and Bit Operations/Compare To Zero  relop=>  OutDataTypeStr=boolean
  Compare To Zero1 : simulink/Logic and Bit Operations/Compare To Zero  relop=>  OutDataTypeStr=boolean
  Compare To Zero2 : simulink/Logic and Bit Operations/Compare To Zero  relop=>  OutDataTypeStr=boolean
  Compare To Zero3 : simulink/Logic and Bit Operations/Compare To Zero  relop=<  OutDataTypeStr=boolean
  Compare To Zero4 : simulink/Logic and Bit Operations/Compare To Zero  relop=<  OutDataTypeStr=boolean
  Compare To Zero5 : simulink/Logic and Bit Operations/Compare To Zero  relop=<  OutDataTypeStr=boolean
  Constant : Constant  Value=6
  Constant1 : Constant  Value=-3
  Display : Display
  Scope12 : Scope  NumInputPorts=4
  Scope6 : Scope  NumInputPorts=6
  Sine Wave Function : Sin  Amplitude=ModulationIndex1  Frequency=ffund*2*pi  Phase=-2*pi/3  SampleTime=0
  Sine Wave Function1 : Sin  Amplitude=ModulationIndex1  Frequency=ffund*2*pi  SampleTime=0
  Sine Wave Function2 : Sin  Amplitude=ModulationIndex1  Frequency=ffund*2*pi  Phase=2*pi/3  SampleTime=0
  Subtract : Sum  Inputs=+-
  Subtract1 : Sum  Inputs=+-
  Subtract2 : Sum  Inputs=+-
  Switch{,1..5} (6 alike) : Switch  Criteria=u2 > Threshold
  Triangle Generator : powerlib_meascontrol/Pulse & Signal Generators/Triangle Generator  Freq=fsw  Phase=Module1Phase  Ts=0
  tag scope: PWMAB=global, PWMAT=global, PWMBB=global, PWMBT=global, PWMCB=global, PWMCT=global
  wires:
  Triangle Generator/1 -> Scope12/1, Subtract2/2, Subtract1/2, Subtract/2
  Compare To Zero2/1 -> Switch2/2
  Subtract1/1 -> Compare To Zero4/1, Compare To Zero1/1
  Subtract/1 -> Compare To Zero3/1, Compare To Zero/1
  Constant/1 -> Switch5/1, Switch4/1, Switch3/1, Switch2/1, Switch1/1, Switch/1
  Compare To Zero/1 -> Switch/2
  Compare To Zero5/1 -> Switch5/2
  Switch3/1 -> [PWMAB], Scope6/4  "ab"
  Switch/1 -> [PWMAT], Display/1, Scope6/1  "at"
  Constant1/1 -> Switch/3, Switch1/3, Switch5/3, Switch4/3, Switch3/3, Switch2/3
  Switch1/1 -> [PWMBT], Scope6/2  "bt"
  Compare To Zero3/1 -> Switch3/2
  Sine Wave Function2/1 -> Scope12/4, Subtract2/1
  Compare To Zero4/1 -> Switch4/2
  Sine Wave Function/1 -> Subtract1/1, Scope12/3
  Compare To Zero1/1 -> Switch1/2
  Subtract2/1 -> Compare To Zero5/1, Compare To Zero2/1
  Switch4/1 -> [PWMBB], Scope6/5  "bb"
  Switch2/1 -> [PWMCT], Scope6/3  "ct"
  Sine Wave Function1/1 -> Scope12/2, Subtract/1
  Switch5/1 -> [PWMCB], Scope6/6  "cb"

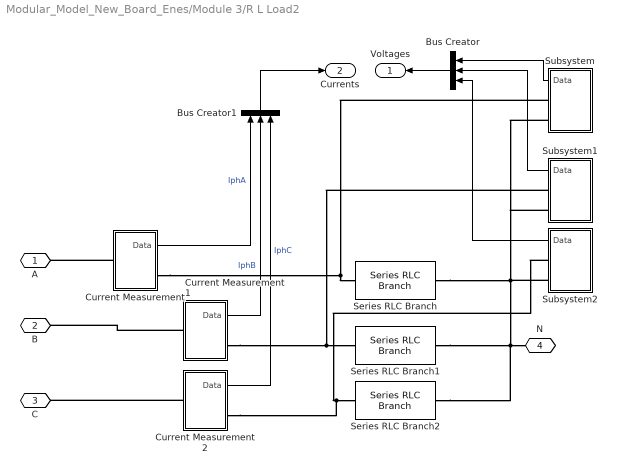
== system Modular_Model_New_Board_Enes/Module 3/R L Load2 ==
  Bus Creator : BusCreator  Inputs=3
  Bus Creator1 : BusCreator  Inputs=3
  Current Measurement : Subsystem
  Current Measurement1 : Subsystem
  Current Measurement2 : Subsystem
  Series RLC Branch : powerlib/Elements/Series RLC Branch  LConnTagsString=__new0  RConnTagsString=__new0  BranchType=RL  Resistance=Rload1  Inductance=Lload1  SetiL0=off  InitialCurrent=0  Capacitance=1e-6  Setx0=off  InitialVoltage=0  Measurements=None
  Series RLC Branch1 : powerlib/Elements/Series RLC Branch  LConnTagsString=__new0  RConnTagsString=__new0  BranchType=RL  Resistance=Rload1  Inductance=Lload1  SetiL0=off  InitialCurrent=0  Capacitance=1e-6  Setx0=off  InitialVoltage=0  Measurements=None
  Series RLC Branch2 : powerlib/Elements/Series RLC Branch  LConnTagsString=__new0  RConnTagsString=__new0  BranchType=RL  Resistance=Rload1  Inductance=Lload1  SetiL0=off  InitialCurrent=0  Capacitance=1e-6  Setx0=off  InitialVoltage=0  Measurements=None
  Subsystem : Subsystem
  Subsystem1 : Subsystem
  Subsystem2 : Subsystem
  A : PMIOPort  Side=Left
  B : PMIOPort  Port=2  Side=Left
  C : PMIOPort  Port=3  Side=Left
  N : PMIOPort  Port=4  Side=Right
  Voltages : Outport
  Currents : Outport  Port=2
  wires:
  Current Measurement/1(Data) -> Bus Creator1/1  "IphA"
  Current Measurement1/1(Data) -> Bus Creator1/2  "IphB"
  Current Measurement2/1(Data) -> Bus Creator1/3  "IphC"
  Bus Creator/1 -> Voltages/1
  Bus Creator1/1 -> Currents/1
  Subsystem/1(Data) -> Bus Creator/1
  Subsystem1/1(Data) -> Bus Creator/2
  Subsystem2/1(Data) -> Bus Creator/3
  connections:
  Current Measurement/LConn1 -- A/RConn1
  Current Measurement1/LConn1 -- B/RConn1
  Current Measurement2/LConn1 -- C/RConn1
  Series RLC Branch1/RConn1 -- Subsystem2/RConn2 -- Subsystem/RConn2 -- Subsystem1/RConn2 -- Series RLC Branch/RConn1 -- N/RConn1 -- Series RLC Branch2/RConn1
  Subsystem/RConn1 -- Current Measurement/RConn1 -- Series RLC Branch/LConn1
  Subsystem1/RConn1 -- Series RLC Branch1/LConn1 -- Current Measurement1/RConn1
  Subsystem2/RConn1 -- Current Measurement2/RConn1 -- Series RLC Branch2/LConn1

== system Modular_Model_New_Board_Enes/Module 3/Subsystem ==
  Voltage Measurement : powerlib/Measurements/Voltage Measurement  PhasorSimulation=off  OutputType=Complex  PSBequivalent=0
  V+ : PMIOPort  Side=Left
  V- : PMIOPort  Port=2  Side=Left
  tag scope: ACap=global
  wires:
  Voltage Measurement/1 -> [ACap]
  connections:
  Voltage Measurement/LConn1 -- V+/RConn1
  Voltage Measurement/LConn2 -- V-/RConn1

== system Modular_Model_New_Board_Enes/Module 3/Subsystem1 ==
  Voltage Measurement : powerlib/Measurements/Voltage Measurement  PhasorSimulation=off  OutputType=Complex  PSBequivalent=0
  V+ : PMIOPort  Side=Left
  V- : PMIOPort  Port=2  Side=Left
  tag scope: BCap=global
  wires:
  Voltage Measurement/1 -> [BCap]
  connections:
  Voltage Measurement/LConn1 -- V+/RConn1
  Voltage Measurement/LConn2 -- V-/RConn1

== system Modular_Model_New_Board_Enes/Module 3/Subsystem2 ==
  Voltage Measurement : powerlib/Measurements/Voltage Measurement  PhasorSimulation=off  OutputType=Complex  PSBequivalent=0
  V+ : PMIOPort  Side=Left
  V- : PMIOPort  Port=2  Side=Left
  tag scope: CCap=global
  wires:
  Voltage Measurement/1 -> [CCap]
  connections:
  Voltage Measurement/LConn1 -- V+/RConn1
  Voltage Measurement/LConn2 -- V-/RConn1

== system Modular_Model_New_Board_Enes/Module 3/Subsystem3 ==
  Voltage Measurement : powerlib/Measurements/Voltage Measurement  PhasorSimulation=off  OutputType=Complex  PSBequivalent=0
  V+ : PMIOPort  Side=Left
  V- : PMIOPort  Port=2  Side=Left
  data : Outport
  wires:
  Voltage Measurement/1 -> data/1
  connections:
  Voltage Measurement/LConn1 -- V+/RConn1
  Voltage Measurement/LConn2 -- V-/RConn1

== system Modular_Model_New_Board_Enes/Module 3/Gate Driver1/Current Measurement ==
  Current Measurement : powerlib/Measurements/Current Measurement  PhasorSimulation=off  OutputType=Complex  PSBequivalent=0
  i- : PMIOPort  Side=Left
  i+ : PMIOPort  Port=2  Side=Right
  Data : Outport
  wires:
  Current Measurement/1 -> Data/1
  connections:
  i-/RConn1 -- Current Measurement/RConn1
  Current Measurement/LConn1 -- i+/RConn1

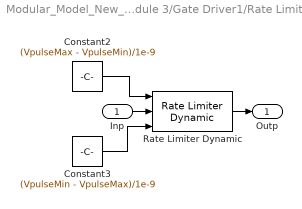
== system Modular_Model_New_Board_Enes/Module 3/Gate Driver1/Rate Limiter2 ==
  Inp : Inport
  Constant2 : Constant  Value=(VpulseMax - VpulseMin)/1e-9
  Constant3 : Constant  Value=(VpulseMin - VpulseMax)/1e-9
  Rate Limiter Dynamic : simulink/Discontinuities/Rate Limiter Dynamic
      settings: SourceProductName=Simulink
  Outp : Outport
  wires:
  Constant3/1 -> Rate Limiter Dynamic/3
  Constant2/1 -> Rate Limiter Dynamic/1
  Inp/1 -> Rate Limiter Dynamic/2
  Rate Limiter Dynamic/1 -> Outp/1

== system Modular_Model_New_Board_Enes/Module 3/Gate Driver1/Subsystem ==
  Voltage Measurement : powerlib/Measurements/Voltage Measurement  PhasorSimulation=off  OutputType=Complex  PSBequivalent=0
  V+ : PMIOPort  Side=Left
  V- : PMIOPort  Port=2  Side=Left
  Data : Outport
  wires:
  Voltage Measurement/1 -> Data/1
  connections:
  Voltage Measurement/LConn1 -- V+/RConn1
  Voltage Measurement/LConn2 -- V-/RConn1

== system Modular_Model_New_Board_Enes/Module 3/Gate Driver2/Current Measurement ==
  Current Measurement : powerlib/Measurements/Current Measurement  PhasorSimulation=off  OutputType=Complex  PSBequivalent=0
  i- : PMIOPort  Side=Left
  i+ : PMIOPort  Port=2  Side=Right
  Data : Outport
  wires:
  Current Measurement/1 -> Data/1
  connections:
  i-/RConn1 -- Current Measurement/RConn1
  Current Measurement/LConn1 -- i+/RConn1

== system Modular_Model_New_Board_Enes/Module 3/Gate Driver2/Rate Limiter2 ==
  Inp : Inport
  Constant2 : Constant  Value=(VpulseMax - VpulseMin)/1e-9
  Constant3 : Constant  Value=(VpulseMin - VpulseMax)/1e-9
  Rate Limiter Dynamic : simulink/Discontinuities/Rate Limiter Dynamic
      settings: SourceProductName=Simulink
  Outp : Outport
  wires:
  Constant3/1 -> Rate Limiter Dynamic/3
  Constant2/1 -> Rate Limiter Dynamic/1
  Inp/1 -> Rate Limiter Dynamic/2
  Rate Limiter Dynamic/1 -> Outp/1

== system Modular_Model_New_Board_Enes/Module 3/Gate Driver2/Subsystem ==
  Voltage Measurement : powerlib/Measurements/Voltage Measurement  PhasorSimulation=off  OutputType=Complex  PSBequivalent=0
  V+ : PMIOPort  Side=Left
  V- : PMIOPort  Port=2  Side=Left
  Data : Outport
  wires:
  Voltage Measurement/1 -> Data/1
  connections:
  Voltage Measurement/LConn1 -- V+/RConn1
  Voltage Measurement/LConn2 -- V-/RConn1

== system Modular_Model_New_Board_Enes/Module 3/Gate Driver3/Current Measurement ==
  Current Measurement : powerlib/Measurements/Current Measurement  PhasorSimulation=off  OutputType=Complex  PSBequivalent=0
  i- : PMIOPort  Side=Left
  i+ : PMIOPort  Port=2  Side=Right
  Data : Outport
  wires:
  Current Measurement/1 -> Data/1
  connections:
  i-/RConn1 -- Current Measurement/RConn1
  Current Measurement/LConn1 -- i+/RConn1

== system Modular_Model_New_Board_Enes/Module 3/Gate Driver3/Rate Limiter2 ==
  Inp : Inport
  Constant2 : Constant  Value=(VpulseMax - VpulseMin)/1e-9
  Constant3 : Constant  Value=(VpulseMin - VpulseMax)/1e-9
  Rate Limiter Dynamic : simulink/Discontinuities/Rate Limiter Dynamic
      settings: SourceProductName=Simulink
  Outp : Outport
  wires:
  Constant3/1 -> Rate Limiter Dynamic/3
  Constant2/1 -> Rate Limiter Dynamic/1
  Inp/1 -> Rate Limiter Dynamic/2
  Rate Limiter Dynamic/1 -> Outp/1

== system Modular_Model_New_Board_Enes/Module 3/Gate Driver3/Subsystem ==
  Voltage Measurement : powerlib/Measurements/Voltage Measurement  PhasorSimulation=off  OutputType=Complex  PSBequivalent=0
  V+ : PMIOPort  Side=Left
  V- : PMIOPort  Port=2  Side=Left
  Data : Outport
  wires:
  Voltage Measurement/1 -> Data/1
  connections:
  Voltage Measurement/LConn1 -- V+/RConn1
  Voltage Measurement/LConn2 -- V-/RConn1

== system Modular_Model_New_Board_Enes/Module 3/Gate Driver4/Current Measurement ==
  Current Measurement : powerlib/Measurements/Current Measurement  PhasorSimulation=off  OutputType=Complex  PSBequivalent=0
  i- : PMIOPort  Side=Left
  i+ : PMIOPort  Port=2  Side=Right
  Data : Outport
  wires:
  Current Measurement/1 -> Data/1
  connections:
  i-/RConn1 -- Current Measurement/RConn1
  Current Measurement/LConn1 -- i+/RConn1

== system Modular_Model_New_Board_Enes/Module 3/Gate Driver4/Rate Limiter2 ==
  Inp : Inport
  Constant2 : Constant  Value=(VpulseMax - VpulseMin)/1e-9
  Constant3 : Constant  Value=(VpulseMin - VpulseMax)/1e-9
  Rate Limiter Dynamic : simulink/Discontinuities/Rate Limiter Dynamic
      settings: SourceProductName=Simulink
  Outp : Outport
  wires:
  Constant3/1 -> Rate Limiter Dynamic/3
  Constant2/1 -> Rate Limiter Dynamic/1
  Inp/1 -> Rate Limiter Dynamic/2
  Rate Limiter Dynamic/1 -> Outp/1

== system Modular_Model_New_Board_Enes/Module 3/Gate Driver4/Subsystem ==
  Voltage Measurement : powerlib/Measurements/Voltage Measurement  PhasorSimulation=off  OutputType=Complex  PSBequivalent=0
  V+ : PMIOPort  Side=Left
  V- : PMIOPort  Port=2  Side=Left
  Data : Outport
  wires:
  Voltage Measurement/1 -> Data/1
  connections:
  Voltage Measurement/LConn1 -- V+/RConn1
  Voltage Measurement/LConn2 -- V-/RConn1

== system Modular_Model_New_Board_Enes/Module 3/Gate Driver5/Current Measurement ==
  Current Measurement : powerlib/Measurements/Current Measurement  PhasorSimulation=off  OutputType=Complex  PSBequivalent=0
  i- : PMIOPort  Side=Left
  i+ : PMIOPort  Port=2  Side=Right
  Data : Outport
  wires:
  Current Measurement/1 -> Data/1
  connections:
  i-/RConn1 -- Current Measurement/RConn1
  Current Measurement/LConn1 -- i+/RConn1

== system Modular_Model_New_Board_Enes/Module 3/Gate Driver5/Rate Limiter1 ==
  Inp : Inport
  Constant2 : Constant  Value=(VpulseMax - VpulseMin)/1e-9
  Constant3 : Constant  Value=(VpulseMin - VpulseMax)/1e-9
  Rate Limiter Dynamic : simulink/Discontinuities/Rate Limiter Dynamic
      settings: SourceProductName=Simulink
  Outp : Outport
  wires:
  Constant3/1 -> Rate Limiter Dynamic/3
  Constant2/1 -> Rate Limiter Dynamic/1
  Inp/1 -> Rate Limiter Dynamic/2
  Rate Limiter Dynamic/1 -> Outp/1

== system Modular_Model_New_Board_Enes/Module 3/Gate Driver5/Subsystem ==
  Voltage Measurement : powerlib/Measurements/Voltage Measurement  PhasorSimulation=off  OutputType=Complex  PSBequivalent=0
  V+ : PMIOPort  Side=Left
  V- : PMIOPort  Port=2  Side=Left
  Data : Outport
  wires:
  Voltage Measurement/1 -> Data/1
  connections:
  Voltage Measurement/LConn1 -- V+/RConn1
  Voltage Measurement/LConn2 -- V-/RConn1

== system Modular_Model_New_Board_Enes/Module 3/Gate Driver6/Current Measurement ==
  Current Measurement : powerlib/Measurements/Current Measurement  PhasorSimulation=off  OutputType=Complex  PSBequivalent=0
  i- : PMIOPort  Side=Left
  i+ : PMIOPort  Port=2  Side=Right
  Data : Outport
  wires:
  Current Measurement/1 -> Data/1
  connections:
  i-/RConn1 -- Current Measurement/RConn1
  Current Measurement/LConn1 -- i+/RConn1

== system Modular_Model_New_Board_Enes/Module 3/Gate Driver6/Rate Limiter2 ==
  Inp : Inport
  Constant2 : Constant  Value=(VpulseMax - VpulseMin)/1e-9
  Constant3 : Constant  Value=(VpulseMin - VpulseMax)/1e-9
  Rate Limiter Dynamic : simulink/Discontinuities/Rate Limiter Dynamic
      settings: SourceProductName=Simulink
  Outp : Outport
  wires:
  Constant3/1 -> Rate Limiter Dynamic/3
  Constant2/1 -> Rate Limiter Dynamic/1
  Inp/1 -> Rate Limiter Dynamic/2
  Rate Limiter Dynamic/1 -> Outp/1

== system Modular_Model_New_Board_Enes/Module 3/Gate Driver6/Subsystem ==
  Voltage Measurement : powerlib/Measurements/Voltage Measurement  PhasorSimulation=off  OutputType=Complex  PSBequivalent=0
  V+ : PMIOPort  Side=Left
  V- : PMIOPort  Port=2  Side=Left
  Data : Outport
  wires:
  Voltage Measurement/1 -> Data/1
  connections:
  Voltage Measurement/LConn1 -- V+/RConn1
  Voltage Measurement/LConn2 -- V-/RConn1

== system Modular_Model_New_Board_Enes/Module 3/R L Load2/Current Measurement ==
  Current Measurement : powerlib/Measurements/Current Measurement  PhasorSimulation=off  OutputType=Complex  PSBequivalent=0
  i- : PMIOPort  Side=Right
  i+ : PMIOPort  Port=2  Side=Left
  Data : Outport
  wires:
  Current Measurement/1 -> Data/1
  connections:
  i-/RConn1 -- Current Measurement/RConn1
  Current Measurement/LConn1 -- i+/RConn1

== system Modular_Model_New_Board_Enes/Module 3/R L Load2/Current Measurement1 ==
  Current Measurement : powerlib/Measurements/Current Measurement  PhasorSimulation=off  OutputType=Complex  PSBequivalent=0
  i- : PMIOPort  Side=Right
  i+ : PMIOPort  Port=2  Side=Left
  Data : Outport
  wires:
  Current Measurement/1 -> Data/1
  connections:
  i-/RConn1 -- Current Measurement/RConn1
  Current Measurement/LConn1 -- i+/RConn1

== system Modular_Model_New_Board_Enes/Module 3/R L Load2/Current Measurement2 ==
  Current Measurement : powerlib/Measurements/Current Measurement  PhasorSimulation=off  OutputType=Complex  PSBequivalent=0
  i- : PMIOPort  Side=Right
  i+ : PMIOPort  Port=2  Side=Left
  Data : Outport
  wires:
  Current Measurement/1 -> Data/1
  connections:
  i-/RConn1 -- Current Measurement/RConn1
  Current Measurement/LConn1 -- i+/RConn1

== system Modular_Model_New_Board_Enes/Module 3/R L Load2/Subsystem ==
  Voltage Measurement : powerlib/Measurements/Voltage Measurement  PhasorSimulation=off  OutputType=Complex  PSBequivalent=0
  V+ : PMIOPort  Side=Right
  V- : PMIOPort  Port=2  Side=Right
  Data : Outport
  wires:
  Voltage Measurement/1 -> Data/1
  connections:
  Voltage Measurement/LConn1 -- V+/RConn1
  Voltage Measurement/LConn2 -- V-/RConn1

== system Modular_Model_New_Board_Enes/Module 3/R L Load2/Subsystem1 ==
  Voltage Measurement : powerlib/Measurements/Voltage Measurement  PhasorSimulation=off  OutputType=Complex  PSBequivalent=0
  V+ : PMIOPort  Side=Right
  V- : PMIOPort  Port=2  Side=Right
  Data : Outport
  wires:
  Voltage Measurement/1 -> Data/1
  connections:
  Voltage Measurement/LConn1 -- V+/RConn1
  Voltage Measurement/LConn2 -- V-/RConn1

== system Modular_Model_New_Board_Enes/Module 3/R L Load2/Subsystem2 ==
  Voltage Measurement : powerlib/Measurements/Voltage Measurement  PhasorSimulation=off  OutputType=Complex  PSBequivalent=0
  V+ : PMIOPort  Side=Right
  V- : PMIOPort  Port=2  Side=Right
  Data : Outport
  wires:
  Voltage Measurement/1 -> Data/1
  connections:
  Voltage Measurement/LConn1 -- V+/RConn1
  Voltage Measurement/LConn2 -- V-/RConn1
